simulink model "UAM_decentralized"  (R2024b)
settings: Solver=VariableStepAuto  StartTime=0.0  StopTime=20  FixedStep=Ts  RelTol=1e-3
InitFcn:
  | UAM_initialization
values from neighbouring files (symbols this model uses):
  eta_b_dot_init = [0;0;0]    [UAM_initialization.m]
  eta_b_init = [0;0;psi0]    [UAM_initialization.m]
  H_b = sym('H_b', [3 3], 'real')    [C_matrix.m]    (also in UAM_initialization.m = diag([1.24, 1.24, 2.48]))
  H_l1 = sym('H_l1', [3 3], 'real')    [C_matrix.m]    (also in C_matrix_manipulator.m; UAM_initialization.m = diag([0, 0, 0]))
  H_l2 = sym('H_l2', [3 3], 'real')    [C_matrix.m]    (also in C_matrix_manipulator.m; UAM_initialization.m = diag([0, 0, 0.0011]))
  H_l3 = sym('H_l3', [3 3], 'real')    [C_matrix.m]    (also in C_matrix_manipulator.m; UAM_initialization.m = diag([0, 0, 1.25e-4]))
  l1 = 0.15    [UAM_initialization.m]
  l2 = 0.05    [UAM_initialization.m]
  m_b = 2.0    (= 2)    [UAM_initialization.m]
  m_l1 = 0    [UAM_initialization.m]
  m_l2 = 0.049    [UAM_initialization.m]
  m_l3 = 0.05    [UAM_initialization.m]
  offset = 0.1    [UAM_initialization.m]
  p_b_dot_init = lin_vel_0'    [UAM_initialization.m]
  p_b_init = pos_0'    [UAM_initialization.m]
  q_dot_init = zeros(3,1)    [UAM_initialization.m]
  q_init = [-pi/2; 0; pi/2]    [UAM_initialization.m]
  Ts = 0.001    [UAM_initialization.m]
undefined symbols (not defined in the file or in its folder): DiscIntNeverNeededParam
libraries: cstblocks x3, simulink x2, simulink_extras x1
settings Model: Creator=giuli  LastModifiedBy=giuli

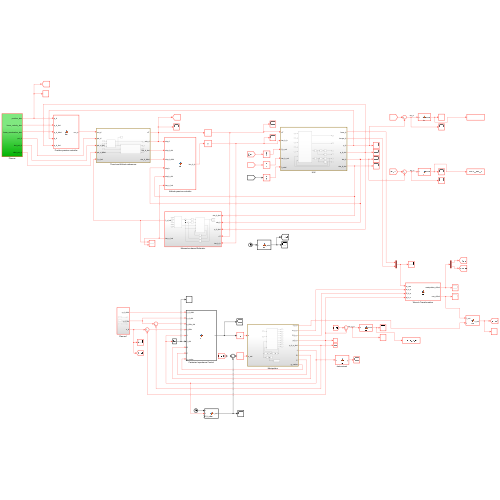
[thumbnail: Simulink's stored preview of the top-level diagram]
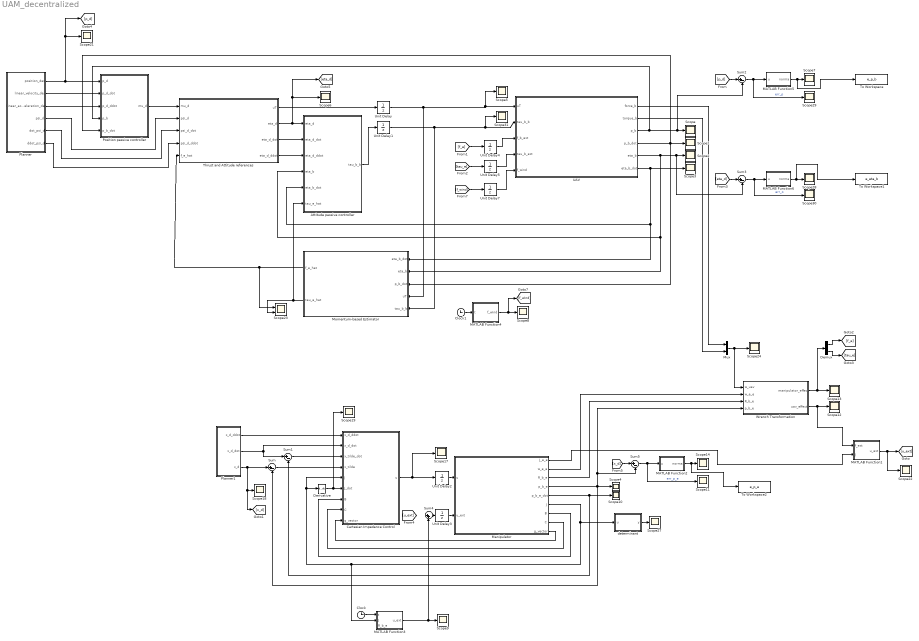
== system UAM_decentralized ==
  Attitude passive controller : MATLAB Function  TreatAsAtomicUnit=on
  Cartesian Impedance Control : MATLAB Function  TreatAsAtomicUnit=on
  Clock : Clock
      settings: Decimation=100
  Clock1 : Clock
      settings: Decimation=100
  Demux : Demux  Outputs=[3 3]
  Derivative : Derivative
  MATLAB Function1 : MATLAB Function  TreatAsAtomicUnit=on
  MATLAB Function2 : MATLAB Function  TreatAsAtomicUnit=on
  MATLAB Function3 : MATLAB Function  TreatAsAtomicUnit=on
  MATLAB Function4 : MATLAB Function  TreatAsAtomicUnit=on
  MATLAB Function5 : MATLAB Function  TreatAsAtomicUnit=on
  MATLAB Function6 : MATLAB Function  TreatAsAtomicUnit=on
  Manipulator : Subsystem
  Momentum-based Estimator : Subsystem
  Mux : Mux  Inputs=[3 3]
  Planner : Subsystem
  Planner1 : Subsystem
  Position passive controller : MATLAB Function  TreatAsAtomicUnit=on
  Scope{,1..14,17..19,21..22,24,27..31} (26 alike) : Scope
  Scope23 : Scope  NumInputPorts=2
  Sum{,1..3,5} (5 alike) : Sum  Inputs=|+-
  Sum4 : Sum  Inputs=|++
  Thrust and Attitude references : Subsystem
  To Workspace : ToWorkspace  VariableName=e_p_b  SampleTime=-1
  To Workspace1 : ToWorkspace  VariableName=e_eta_b  SampleTime=-1
  To Workspace2 : ToWorkspace  VariableName=e_p_e  SampleTime=-1
  UAV : Subsystem
  Unit Delay : UnitDelay  InitialCondition=m_b*9.81  SampleTime=Ts  HasFrameUpgradeWarning=on
  Unit Delay{1..5} (5 alike) : UnitDelay  SampleTime=Ts  HasFrameUpgradeWarning=on
  Unit Delay7 : UnitDelay  SampleTime=-1  HasFrameUpgradeWarning=on
  Wrench Transformation : MATLAB Function  TreatAsAtomicUnit=on
  determinant : MATLAB Function  TreatAsAtomicUnit=on
  wires:
  Attitude passive controller/1(tau_b_b) -> Unit Delay1/1
  [f_e] -> Unit Delay4/1
  [tau_e] -> Unit Delay5/1
  Thrust and Attitude references/4(eta_d_ddot) -> Attitude passive controller/3(eta_d_ddot)
  Thrust and Attitude references/1(uT) -> Unit Delay/1
  Thrust and Attitude references/3(eta_d_dot) -> Attitude passive controller/2(eta_d_dot)
  Thrust and Attitude references/2(eta_d) -> Attitude passive controller/1(eta_d), Scope6/1, [eta_d]
  Position passive controller/1(mu_d) -> Thrust and Attitude references/1(mu_d)
  Planner/1(position_des) -> Scope21/1, [p_d], Position passive controller/1(p_d)
  Planner/2(linear_velocity_des) -> Position passive controller/2(p_d_dot)
  Planner/3(linear_acceleration_des) -> Position passive controller/3(p_d_ddot)
  Planner/4(psi_d) -> Thrust and Attitude references/2(psi_d)
  Planner/5(dot_psi_d) -> Thrust and Attitude references/3(psi_d_dot)
  Planner/6(ddot_psi_d) -> Thrust and Attitude references/4(psi_d_ddot)
  Momentum-based Estimator/2(tau_e_hat) -> Scope23/2, Attitude passive controller/6(tau_e_hat)
  Momentum-based Estimator/1(f_e_hat) -> Thrust and Attitude references/5(f_e_hat), Scope23/1
  UAV/6(eta_b_dot) -> Attitude passive controller/5(eta_b_dot), Momentum-based Estimator/1(eta_b_dot), Scope3/1
  UAV/5(eta_b) -> Sum3/2, Scope2/1, Attitude passive controller/4(eta_b), Momentum-based Estimator/2(eta_b)
  UAV/4(p_b_dot) -> Position passive controller/5(p_b_dot), Scope1/1, Momentum-based Estimator/3(p_b_dot)
  UAV/3(p_b) -> Position passive controller/4(p_b), Scope/1, Sum2/2
  Sum/1 -> Cartesian Impedance Control/4(x_tilde)
  Manipulator/9(g_vector) -> Cartesian Impedance Control/9(g_vector)
  MATLAB Function3/1(u_ext) -> Sum4/2, Scope9/1
  Manipulator/8(C) -> Cartesian Impedance Control/8(C)
  Sum1/1 -> Cartesian Impedance Control/3(x_tilde_dot)
  Unit Delay2/1 -> Manipulator/1(u)
  Clock/1 -> MATLAB Function3/1(t)
  Manipulator/4(p_b_e) -> Wrench Transformation/4(p_b_e), Sum5/2, Scope4/1, Sum/2
  Manipulator/5(p_b_e_dot) -> Scope10/1, Sum1/2
  Manipulator/7(B) -> Cartesian Impedance Control/7(B)
  Derivative/1 -> Scope19/1, Cartesian Impedance Control/6(J_dot)
  MATLAB Function1/1(u_ext) -> [u_ext], Scope22/1
  Demux/1 -> [f_e]
  Unit Delay4/1 -> UAV/3(f_b_ext)
  UAV/1(force_b) -> Mux/1
  UAV/2(torque_b) -> Mux/2
  Manipulator/6(J) -> determinant/1(u), Derivative/1, Cartesian Impedance Control/5(J), MATLAB Function3/2(J)
  Planner1/3(x_d) -> [x_d], Scope18/1, Sum/1
  Planner1/2(x_d_dot) -> Sum1/1, Cartesian Impedance Control/2(x_d_dot)
  Planner1/1(x_d_ddot) -> Cartesian Impedance Control/1(x_d_ddot)
  Cartesian Impedance Control/1(u) -> Unit Delay2/1, Scope17/1
  determinant/1(y) -> Scope27/1
  Unit Delay/1 -> Scope5/1, UAV/1(uT), Momentum-based Estimator/4(uT)
  Unit Delay1/1 -> Scope31/1, UAV/2(tau_b_b), Momentum-based Estimator/5(tau_b_b)
  Wrench Transformation/1(manipulator_effect) -> Demux/1, Scope13/1
  Wrench Transformation/2(uav_effect) -> MATLAB Function1/1(f_ext), Scope12/1
  Demux/2 -> [tau_e]
  Unit Delay5/1 -> UAV/4(tau_b_ext)
  [p_d] -> Sum2/1
  Sum2/1 -> Scope29/1, MATLAB Function5/1(u)  "err_p"
  MATLAB Function5/1(norma) -> To Workspace/1, Scope7/1
  MATLAB Function6/1(norma) -> To Workspace1/1, Scope28/1
  Sum3/1 -> Scope30/1, MATLAB Function6/1(u)  "err_o"
  [eta_d] -> Sum3/1
  [x_d] -> Sum5/1
  Sum5/1 -> Scope11/1, MATLAB Function2/1(u)  "err_p_e"
  MATLAB Function2/1(norma) -> To Workspace2/1, Scope14/1
  Manipulator/2(w_e_e) -> Wrench Transformation/2(w_e_e)
  Manipulator/3(R_b_e) -> Wrench Transformation/3(R_b_e)
  Manipulator/1(J_e_e) -> MATLAB Function1/2(J)
  Mux/1 -> Wrench Transformation/1(w_uav), Scope24/1
  Clock1/1 -> MATLAB Function4/1(t)
  MATLAB Function4/1(f_wind) -> [f_wind], Scope8/1
  Sum4/1 -> Unit Delay3/1
  Unit Delay7/1 -> UAV/5(f_wind)
  [f_wind] -> Unit Delay7/1
  Unit Delay3/1 -> Manipulator/2(u_ext)

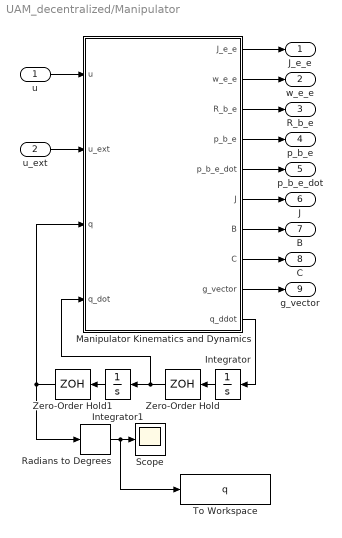
== system UAM_decentralized/Manipulator ==
  u : Inport
  u_ext : Inport  Port=2
  Integrator : Integrator  InitialCondition=q_dot_init
  Integrator1 : Integrator  InitialCondition=q_init
  Manipulator Kinematics and Dynamics : MATLAB Function  TreatAsAtomicUnit=on
  Radians to Degrees : simulink_extras/Transformations/Radians to Degrees
  Scope : Scope
  To Workspace : ToWorkspace  VariableName=q  SampleTime=-1
  Zero-Order Hold : ZeroOrderHold  SampleTime=Ts
  Zero-Order Hold1 : ZeroOrderHold  SampleTime=Ts
  J_e_e : Outport
  w_e_e : Outport  Port=2
  R_b_e : Outport  Port=3
  p_b_e : Outport  Port=4
  p_b_e_dot : Outport  Port=5
  J : Outport  Port=6
  B : Outport  Port=7
  C : Outport  Port=8
  g_vector : Outport  Port=9
  wires:
  u_ext/1 -> Manipulator Kinematics and Dynamics/2(u_ext)
  Manipulator Kinematics and Dynamics/9(g_vector) -> g_vector/1
  u/1 -> Manipulator Kinematics and Dynamics/1(u)
  Manipulator Kinematics and Dynamics/6(J) -> J/1
  Manipulator Kinematics and Dynamics/7(B) -> B/1
  Manipulator Kinematics and Dynamics/8(C) -> C/1
  Manipulator Kinematics and Dynamics/3(R_b_e) -> R_b_e/1
  Manipulator Kinematics and Dynamics/4(p_b_e) -> p_b_e/1
  Manipulator Kinematics and Dynamics/5(p_b_e_dot) -> p_b_e_dot/1
  Integrator/1 -> Zero-Order Hold/1
  Manipulator Kinematics and Dynamics/10(q_ddot) -> Integrator/1
  Integrator1/1 -> Zero-Order Hold1/1
  Radians to Degrees/1 -> To Workspace/1, Scope/1
  Zero-Order Hold1/1 -> Manipulator Kinematics and Dynamics/3(q), Radians to Degrees/1
  Zero-Order Hold/1 -> Integrator1/1, Manipulator Kinematics and Dynamics/4(q_dot)
  Manipulator Kinematics and Dynamics/2(w_e_e) -> w_e_e/1
  Manipulator Kinematics and Dynamics/1(J_e_e) -> J_e_e/1

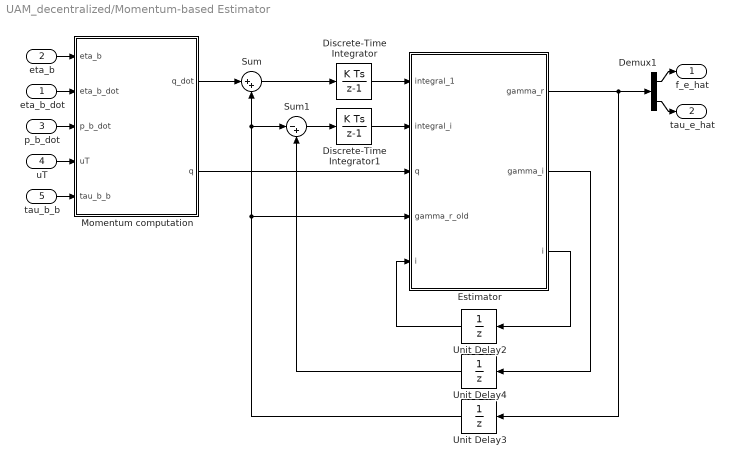
== system UAM_decentralized/Momentum-based Estimator ==
  eta_b_dot : Inport
  eta_b : Inport  Port=2
  p_b_dot : Inport  Port=3
  uT : Inport  Port=4
  tau_b_b : Inport  Port=5
  Demux1 : Demux  Outputs=[3 3]
  Discrete-Time Integrator : DiscreteIntegrator  SampleTime=Ts  ICPrevOutput=DiscIntNeverNeededParam  ICPrevScaledInput=DiscIntNeverNeededParam
  Discrete-Time Integrator1 : DiscreteIntegrator  SampleTime=Ts  ICPrevOutput=DiscIntNeverNeededParam  ICPrevScaledInput=DiscIntNeverNeededParam
  Estimator : MATLAB Function  TreatAsAtomicUnit=on
  Momentum computation : MATLAB Function  TreatAsAtomicUnit=on
  Sum : Sum  Inputs=|++
  Sum1 : Sum  Inputs=|-+
  Unit Delay2 : UnitDelay  SampleTime=-1  HasFrameUpgradeWarning=on
  Unit Delay3 : UnitDelay  SampleTime=-1  HasFrameUpgradeWarning=on
  Unit Delay4 : UnitDelay  SampleTime=-1  HasFrameUpgradeWarning=on
  f_e_hat : Outport
  tau_e_hat : Outport  Port=2
  wires:
  Discrete-Time Integrator/1 -> Estimator/1(integral_1)
  Unit Delay2/1 -> Estimator/5("i ")
  Discrete-Time Integrator1/1 -> Estimator/2(integral_i)
  Unit Delay4/1 -> Sum1/2
  eta_b/1 -> Momentum computation/1(eta_b)
  Demux1/1 -> f_e_hat/1
  Estimator/1(gamma_r) -> Demux1/1, Unit Delay3/1
  Estimator/3(i) -> Unit Delay2/1
  Unit Delay3/1 -> Estimator/4(gamma_r_old), Sum/2, Sum1/1
  Estimator/2(gamma_i) -> Unit Delay4/1
  Sum1/1 -> Discrete-Time Integrator1/1
  Sum/1 -> Discrete-Time Integrator/1
  Momentum computation/1(q_dot) -> Sum/1
  eta_b_dot/1 -> Momentum computation/2(eta_b_dot)
  p_b_dot/1 -> Momentum computation/3(p_b_dot)
  uT/1 -> Momentum computation/4(uT)
  tau_b_b/1 -> Momentum computation/5(tau_b_b)
  Demux1/2 -> tau_e_hat/1
  Momentum computation/2(q) -> Estimator/3(q)

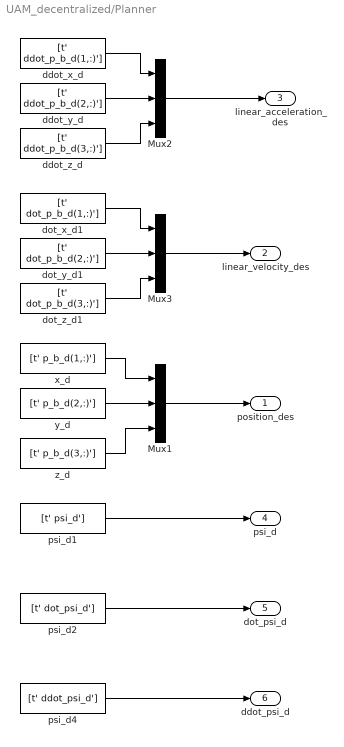
== system UAM_decentralized/Planner ==
  Mux1 : Mux  Inputs=3
  Mux2 : Mux  Inputs=3
  Mux3 : Mux  Inputs=3
  ddot_x_d : FromWorkspace  VariableName=[t' ddot_p_b_d(1,:)']  SampleTime=Ts
  ddot_y_d : FromWorkspace  VariableName=[t' ddot_p_b_d(2,:)']  SampleTime=Ts
  ddot_z_d : FromWorkspace  VariableName=[t' ddot_p_b_d(3,:)']  SampleTime=Ts
  dot_x_d1 : FromWorkspace  VariableName=[t' dot_p_b_d(1,:)']  SampleTime=Ts
  dot_y_d1 : FromWorkspace  VariableName=[t' dot_p_b_d(2,:)']  SampleTime=Ts
  dot_z_d1 : FromWorkspace  VariableName=[t' dot_p_b_d(3,:)']  SampleTime=Ts
  psi_d1 : FromWorkspace  VariableName=[t' psi_d']  SampleTime=Ts
  psi_d2 : FromWorkspace  VariableName=[t' dot_psi_d']  SampleTime=Ts
  psi_d4 : FromWorkspace  VariableName=[t' ddot_psi_d']  SampleTime=Ts
  x_d : FromWorkspace  VariableName=[t' p_b_d(1,:)']  SampleTime=Ts
  y_d : FromWorkspace  VariableName=[t' p_b_d(2,:)']  SampleTime=Ts
  z_d : FromWorkspace  VariableName=[t' p_b_d(3,:)']  SampleTime=Ts
  position_des : Outport
  linear_velocity_des : Outport  Port=2
  linear_acceleration_des : Outport  Port=3
  psi_d : Outport  Port=4
  dot_psi_d : Outport  Port=5
  ddot_psi_d : Outport  Port=6
  wires:
  y_d/1 -> Mux1/2
  z_d/1 -> Mux1/3
  x_d/1 -> Mux1/1
  ddot_y_d/1 -> Mux2/2
  ddot_z_d/1 -> Mux2/3
  ddot_x_d/1 -> Mux2/1
  Mux2/1 -> linear_acceleration_des/1
  Mux1/1 -> position_des/1
  dot_y_d1/1 -> Mux3/2
  dot_z_d1/1 -> Mux3/3
  dot_x_d1/1 -> Mux3/1
  Mux3/1 -> linear_velocity_des/1
  psi_d1/1 -> psi_d/1
  psi_d2/1 -> dot_psi_d/1
  psi_d4/1 -> ddot_psi_d/1

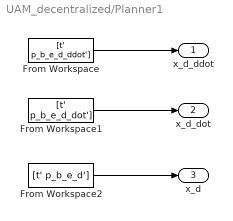
== system UAM_decentralized/Planner1 ==
  From Workspace : FromWorkspace  VariableName=[t' p_b_e_d_ddot']  SampleTime=Ts
  From Workspace1 : FromWorkspace  VariableName=[t' p_b_e_d_dot']  SampleTime=Ts
  From Workspace2 : FromWorkspace  VariableName=[t' p_b_e_d']  SampleTime=Ts
  x_d_ddot : Outport
  x_d_dot : Outport  Port=2
  x_d : Outport  Port=3
  wires:
  From Workspace/1 -> x_d_ddot/1
  From Workspace2/1 -> x_d/1
  From Workspace1/1 -> x_d_dot/1

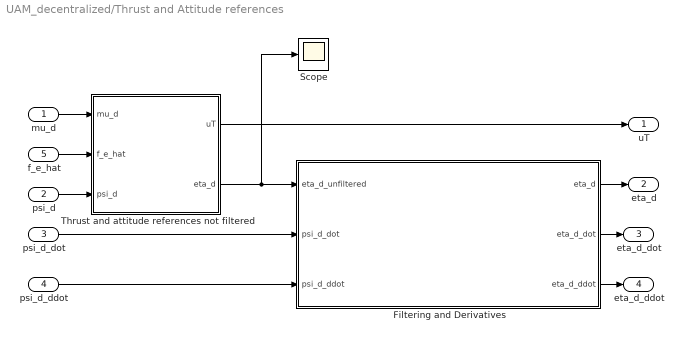
== system UAM_decentralized/Thrust and Attitude references ==
  mu_d : Inport
  psi_d : Inport  Port=2
  psi_d_dot : Inport  Port=3
  psi_d_ddot : Inport  Port=4
  f_e_hat : Inport  Port=5
  Filtering and Derivatives : Subsystem
  Scope : Scope
  Thrust and attitude references not filtered : MATLAB Function  TreatAsAtomicUnit=on
  uT : Outport
  eta_d : Outport  Port=2
  eta_d_dot : Outport  Port=3
  eta_d_ddot : Outport  Port=4
  wires:
  Thrust and attitude references not filtered/2(eta_d) -> Scope/1, Filtering and Derivatives/1(eta_d_unfiltered)
  psi_d_dot/1 -> Filtering and Derivatives/2(psi_d_dot)
  Filtering and Derivatives/3(eta_d_ddot) -> eta_d_ddot/1
  mu_d/1 -> Thrust and attitude references not filtered/1(mu_d)
  Filtering and Derivatives/1(eta_d) -> eta_d/1
  psi_d_ddot/1 -> Filtering and Derivatives/3(psi_d_ddot)
  Filtering and Derivatives/2(eta_d_dot) -> eta_d_dot/1
  f_e_hat/1 -> Thrust and attitude references not filtered/2(f_e_hat)
  psi_d/1 -> Thrust and attitude references not filtered/3(psi_d)
  Thrust and attitude references not filtered/1(uT) -> uT/1

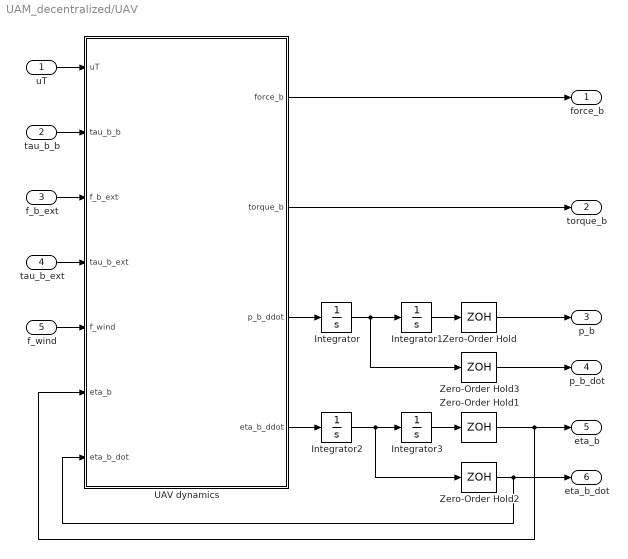
== system UAM_decentralized/UAV ==
  uT : Inport
  tau_b_b : Inport  Port=2
  f_b_ext : Inport  Port=3
  tau_b_ext : Inport  Port=4
  f_wind : Inport  Port=5
  Integrator : Integrator  InitialCondition=p_b_dot_init
  Integrator1 : Integrator  InitialCondition=p_b_init
  Integrator2 : Integrator  InitialCondition=eta_b_dot_init
  Integrator3 : Integrator  InitialCondition=eta_b_init
  UAV dynamics : MATLAB Function  TreatAsAtomicUnit=on
  Zero-Order Hold{,1..3} (4 alike) : ZeroOrderHold  SampleTime=Ts
  force_b : Outport
  torque_b : Outport  Port=2
  p_b : Outport  Port=3
  p_b_dot : Outport  Port=4
  eta_b : Outport  Port=5
  eta_b_dot : Outport  Port=6
  wires:
  Integrator2/1 -> Integrator3/1, Zero-Order Hold2/1
  Zero-Order Hold2/1 -> eta_b_dot/1, UAV dynamics/7(eta_b_dot)
  Integrator3/1 -> Zero-Order Hold1/1
  tau_b_ext/1 -> UAV dynamics/4(tau_b_ext)
  Zero-Order Hold3/1 -> p_b_dot/1
  Integrator/1 -> Integrator1/1, Zero-Order Hold3/1
  UAV dynamics/3(p_b_ddot) -> Integrator/1
  uT/1 -> UAV dynamics/1(uT)
  UAV dynamics/4(eta_b_ddot) -> Integrator2/1
  Integrator1/1 -> Zero-Order Hold/1
  Zero-Order Hold1/1 -> eta_b/1, UAV dynamics/6(eta_b)
  Zero-Order Hold/1 -> p_b/1
  tau_b_b/1 -> UAV dynamics/2(tau_b_b)
  f_b_ext/1 -> UAV dynamics/3(f_b_ext)
  UAV dynamics/1(force_b) -> force_b/1
  UAV dynamics/2(torque_b) -> torque_b/1
  f_wind/1 -> UAV dynamics/5(f_wind)

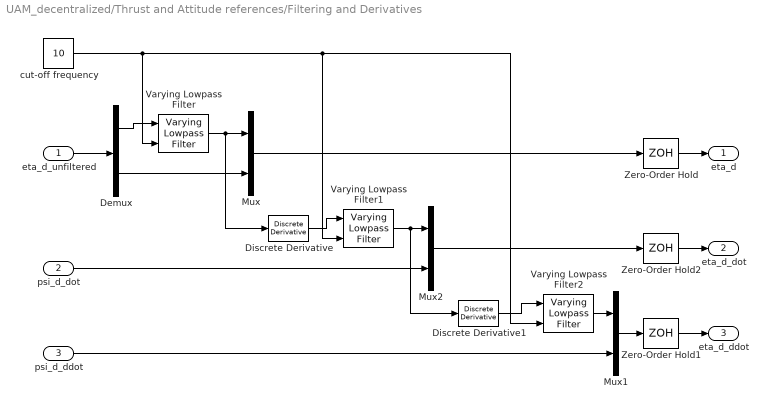
== system UAM_decentralized/Thrust and Attitude references/Filtering and Derivatives ==
  eta_d_unfiltered : Inport
  psi_d_dot : Inport  Port=2
  psi_d_ddot : Inport  Port=3
  Demux : Demux  Outputs=[2 1]
  Discrete Derivative : simulink/Discrete/Discrete Derivative  gainval=1.0  ICPrevScaledInput=0.0  OutMin=[]  OutMax=[]  OutDataType=fixdt(1, 16)  OutScaling=2^-10  DoSatur=off
  Discrete Derivative1 : simulink/Discrete/Discrete Derivative  gainval=1.0  ICPrevScaledInput=0.0  OutMin=[]  OutMax=[]  OutDataType=fixdt(1, 16)  OutScaling=2^-10  DoSatur=off
  Mux : Mux  Inputs=[2 1]
  Mux1 : Mux  Inputs=[2 1]
  Mux2 : Mux  Inputs=[2 1]
  Varying Lowpass Filter : cstblocks/Linear Parameter Varying/Varying Lowpass Filter  N=1
  Varying Lowpass Filter1 : cstblocks/Linear Parameter Varying/Varying Lowpass Filter  N=1
  Varying Lowpass Filter2 : cstblocks/Linear Parameter Varying/Varying Lowpass Filter  N=1
  Zero-Order Hold : ZeroOrderHold  SampleTime=Ts
  Zero-Order Hold1 : ZeroOrderHold  SampleTime=Ts
  Zero-Order Hold2 : ZeroOrderHold  SampleTime=Ts
  cut-off frequency : Constant  Value=10
  eta_d : Outport
  eta_d_dot : Outport  Port=2
  eta_d_ddot : Outport  Port=3
  wires:
  Mux/1 -> Zero-Order Hold/1
  Mux1/1 -> Zero-Order Hold1/1
  Mux2/1 -> Zero-Order Hold2/1
  eta_d_unfiltered/1 -> Demux/1
  psi_d_ddot/1 -> Mux1/2
  Varying Lowpass Filter1/1 -> Discrete Derivative1/1, Mux2/1
  Demux/2 -> Mux/2
  Demux/1 -> Varying Lowpass Filter/1
  Varying Lowpass Filter/1 -> Discrete Derivative/1, Mux/1
  cut-off frequency/1 -> Varying Lowpass Filter/2, Varying Lowpass Filter2/2, Varying Lowpass Filter1/2
  psi_d_dot/1 -> Mux2/2
  Discrete Derivative/1 -> Varying Lowpass Filter1/1
  Discrete Derivative1/1 -> Varying Lowpass Filter2/1
  Varying Lowpass Filter2/1 -> Mux1/1
  Zero-Order Hold/1 -> eta_d/1
  Zero-Order Hold1/1 -> eta_d_ddot/1
  Zero-Order Hold2/1 -> eta_d_dot/1

== matlab function UAM_decentralized/Momentum-based Estimator/Momentum computation ==
  data: q_dot output; eta_b input; q output; eta_b_dot input; p_b_dot input; uT input; tau_b_b input; m_b parameter; H_b parameter
function [q_dot,q] = fcn(eta_b, eta_b_dot, p_b_dot, uT, tau_b_b,  m_b, H_b)

% parameters
g = 9.81;
e3 = [0;0;1];

%% Extracting variables
% Euler angles
phi = eta_b(1);    % Roll angle
theta = eta_b(2);  % Pitch angle
psi = eta_b(3);    % Yaw angle

phi_dot = eta_b_dot(1);   
theta_dot = eta_b_dot(2);  
%psi_dot = eta_b_dot(3);    

%% Rotation Matrices and Angular Velocity Mapping
% Individual Rotation Matrices
% Rotation about X-axis (Roll)
Rx = [1,           0,          0;
      0, cos(phi), -sin(phi);
      0, sin(phi),  cos(phi)];

% Rotation about Y-axis (Pitch)
Ry = [cos(theta),  0, sin(theta);
      0,           1,          0;
     -sin(theta),  0, cos(theta)];

% Rotation about Z-axis (Yaw)
Rz = [cos(psi), -sin(psi), 0;
      sin(psi),  cos(psi), 0;
      0,         0,         1];

% Combined Rotation Matrix R_b (from UAV body frame to Inertial frame)
% Using Z-Y-X Euler angle convention (Yaw-Pitch-Roll)
R_b = Rz * Ry * Rx;

% mapping between time derivative of eta_b into UAV angular velocity omega_b_b expressed wrt Sigma_b
Q = [   1     0           -sin(theta);
        0     cos(phi)    cos(theta)*sin(phi);
        0     -sin(phi)   cos(theta)*cos(phi)];

Q_dot = [ 0,     0,                     -cos(theta)*theta_dot;
          0,    -sin(phi)*phi_dot,     -sin(theta)*sin(phi)*theta_dot + cos(theta)*cos(phi)*phi_dot;
          0,    -cos(phi)*phi_dot,     -sin(theta)*cos(phi)*theta_dot - cos(theta)*sin(phi)*phi_dot ];

%% Dynamic Matrices
M = Q' * H_b * Q;    % inertia matrix
C = Q' * skew(Q * eta_b_dot) * H_b * Q + Q' * H_b * Q_dot;    % Coriolis matrix

%% Generalized momentum q
q = [m_b * p_b_dot;
    M * eta_b_dot];

q_dot = [m_b*g*e3 - uT*R_b*e3;
        C'*eta_b_dot + Q'*tau_b_b];

end

function S = skew(v)
if(numel(v)~= 1)
S= [0 -v(3) v(2); 
    v(3) 0 -v(1);
    -v(2) v(1) 0];
else
S= zeros(3);
end
end

== matlab function UAM_decentralized/Momentum-based Estimator/Estimator ==
  data: gamma_r output; integral_1 input; gamma_i output; integral_i input; q input; gamma_r_old input; i output; i input; K parameter
function [gamma_r, gamma_i, i] = fcn(integral_1, integral_i, q, gamma_r_old,i,  K)

r = 2;

gamma_i = zeros(6,1);
gamma_r = gamma_r_old;

if i == 0   % first step
    i = i+1;
    gamma_i = K(1) * (q - integral_1);
else 
    i = i+1;
    gamma_i = K(i) * integral_i;
    if i == r
        gamma_r = gamma_i;  % final step
        i = 0;  % to reset
    end
end

== matlab function UAM_decentralized/MATLAB Function3 ==
  data: t input; J input; u_ext output; R_b_e input
function u_ext = fcn(t,J,R_b_e)
% A = 1;
% omega = pi/2;
% 
% if t <= 10
%     wind = A*sin(omega*t);
% 
%     if wind >= 0
%         f_ext = [wind; zeros(2,1)];
%     else
%         f_ext = zeros(3,1);
%     end
% else
%     f_ext = zeros(3,1);
% end
% 
% f_ext = R_b_e * [0; 0; 1];

f_wall = [-0.5;0;0];
u_ext = J' * f_wall;

== matlab function UAM_decentralized/MATLAB Function4 ==
  data: t input; f_wind output
function f_wind = fcn(t)
A = 1;
omega = pi/2;

if t <= 10
    wind = A*sin(omega*t);

    if wind >= 0
        f_ext = [wind; zeros(2,1)];
    else
        f_ext = zeros(3,1);
    end
else
    f_ext = zeros(3,1);
end

f_wind = [f_ext(1:3)]; 


% % u_ext = J' * f_ext;

== matlab function UAM_decentralized/Manipulator/Manipulator Kinematics and Dynamics ==
  data: J_e_e output; w_e_e output; R_b_e output; p_b_e output; p_b_e_dot output; J output; B output; C output; g_vector output; u input; u_ext input; q input; q_ddot output; q_dot input; m_l1 parameter; m_l2 parameter; m_l3 parameter; l1 parameter; l2 parameter; H_l1 parameter; H_l2 parameter; H_l3 parameter; offset parameter
function [J_e_e,w_e_e,R_b_e, p_b_e,p_b_e_dot,  J,B,C,g_vector,  q_ddot] = fcn(u, u_ext, q,q_dot, m_l1, m_l2, m_l3, l1, l2, H_l1, H_l2, H_l3, offset) % m_b, H_b

% Parameters
g = 9.81;       % gravity acceleration value
e3 = [0;0;1];   % selecting vector

%% State Variables from Generalized Joints Vector (csi)
% % Extracting components of the generalized state vector 'csi'
% p_b = csi(1:3);    % Position of UAV body frame origin in inertial frame
% eta_b = csi(4:6);  % Euler angles (Yaw, Pitch, Roll) of UAV body frame
% q = csi(7:9);      % Manipulator joint angles
% 
% % Euler angles
% phi = eta_b(1);    % Roll angle
% theta = eta_b(2);  % Pitch angle
% psi = eta_b(3);    % Yaw angle

%% UAV Kinematics: Rotation Matrices and Angular Velocity Mapping
% % Individual Rotation Matrices
% % Rotation about X-axis (Roll)
% Rx = [1,           0,          0;
%       0, cos(phi), -sin(phi);
%       0, sin(phi),  cos(phi)];
% 
% % Rotation about Y-axis (Pitch)
% Ry = [cos(theta),  0, sin(theta);
%       0,           1,          0;
%      -sin(theta),  0, cos(theta)];
% 
% % Rotation about Z-axis (Yaw)
% Rz = [cos(psi), -sin(psi), 0;
%       sin(psi),  cos(psi), 0;
%       0,         0,         1];
% 
% % Combined Rotation Matrix R_b (from UAV body frame to Inertial frame)
% % Using Z-Y-X Euler angle convention (Yaw-Pitch-Roll)
% R_b = Rz * Ry * Rx;
% 
% % mapping between time derivative of eta_b into UAV angular velocity omega_b_b expressed wrt Sigma_b
% Q = [   1     0           -sin(theta);
%         0     cos(phi)    cos(theta)*sin(phi);
%         0     -sin(phi)   cos(theta)*cos(phi)];    % It's easier to compute first Q
% 
% % T_b matrix: Maps Euler angle rates (phi_dot) to body angular velocity (omega_b)
% % omega_b = T_b * phi_dot
% T_b = R_b * Q;        % it's easier this way
% 
% % Q = R_b' * T_b;     
% 
% % Ab: Homogeneous transformation matrix from Inertial frame to UAV Body frame
% A_b = [R_b,   p_b;
%       0 0 0, 1];


%% Manipulator Direct Kinematics (Relative to UAV Body Frame)
% Static Transformation to take into account the offset between UAV and Manipulator

R_b_0 = [1,           0,          0;
        0, cos(pi/2), -sin(pi/2);
        0, sin(pi/2),  cos(pi/2)];  % rotation of pi/2 about x-axis


T_b_0 = [   R_b_0, [0;0;-offset];      % translation along zb
            0,   0,   0,   1];

% D-H parameters for the manipulator
a = [0, l1, l2];
d = [0, 0, 0];
alpha = [pi/2, -pi/2, 0];

% Standard DH transformation matrix A(alpha, a, d, theta) - here theta is q_i
DH_matrix = @(alpha_i, a_i, d_i, q_i) ...
    [cos(q_i), -sin(q_i)*cos(alpha_i),  sin(q_i)*sin(alpha_i),  a_i*cos(q_i);
     sin(q_i),  cos(q_i)*cos(alpha_i), -cos(q_i)*sin(alpha_i),  a_i*sin(q_i);
     0,         sin(alpha_i),          cos(alpha_i),           d_i;
     0,         0,                     0,                      1];

A_0_1 = DH_matrix(alpha(1), a(1), d(1), q(1));
A_1_2 = DH_matrix(alpha(2), a(2), d(2), q(2));
A_2_3 = DH_matrix(alpha(3), a(3), d(3), q(3));

% Transformations from manipulator base frame (Frame 0) to each link frame
T_0_0 = eye(4); % Transformation from Frame 0 to Frame 0
T_0_1 = A_0_1;  % Transformation from Frame 0 to Frame 1
T_0_2 = A_0_1 * A_1_2; % Transformation from Frame 0 to Frame 2
T_0_3 = A_0_1 * A_1_2 * A_2_3; % Transformation from Frame 0 to Frame 3

R_0_0 = T_0_0(1:3, 1:3); p_0_0 = T_0_0(1:3, 4);
R_0_1 = T_0_1(1:3, 1:3); p_0_1 = T_0_1(1:3, 4);
R_0_2 = T_0_2(1:3, 1:3); p_0_2 = T_0_2(1:3, 4);

% Rotation about the y-axis
R_3_e = [cos(pi/2),  0, sin(pi/2);
        0,           1,          0;
        -sin(pi/2),  0, cos(pi/2)];
% To align the z-axis to the approach axis
T_3_e = [R_3_e,         zeros(3,1);
         zeros(1,3),    1];

T_0_e = T_0_3 * T_3_e;

p_0_e = T_0_e(1:3, 4);
R_0_e = T_0_e(1:3, 1:3);

% Direct kinematic of the Manipulator from UAV body frame to end-effector frame
A_b_e = T_b_0 * T_0_3 * T_3_e;

% Extract position of end-effector frame origin in UAV body frame (p_b_e)
% p_e^b is position vector of the origin of end-effector frame wrt Sigma_b 
p_b_e = A_b_e(1:3, 4);

R_b_e = A_b_e(1:3, 1:3);

%% Absolute Pose of the End-Effector
% % A_e: Absolute homogeneous transformation matrix of the end-effector (in Inertial frame)
% A_e = A_b * A_b_e;
% 
% R_e = A_e(1:3, 1:3);
% 
% % Extract p_e (position of end-effector in inertial frame)
% p_e = A_e(1:3, 4); % This is p_e from x = [p_b^T, eta_b^T, p_e^T]^T 
% 
% x = [p_b; eta_b; p_e];

%% Manipulator Jacobian (in manipulator 0 frame)
% For revolute joints
% JPi = z_{i-1} X (p_e - p_{i-1})
% JOi = z_{i-1}

% z_{i-1} is the third column of the rotation matrix R_0_{i-1}
z_0 = R_0_0(:, 3);
z_1 = R_0_1(:, 3);
z_2 = R_0_2(:, 3);

% Manipulator Translational Jacobian (J_P_0_e) for End-Effector in Frame 0
J_P_0_e = zeros(3,3);
J_P_0_e(:,1) = skew(z_0) * (p_0_e - p_0_0);
J_P_0_e(:,2) = skew(z_1) * (p_0_e - p_0_1);
J_P_0_e(:,3) = skew(z_2) * (p_0_e - p_0_2);

% Manipulator Rotational Jacobian (J_O_0_e) for End-Effector in Frame 0
J_O_0_e = zeros(3,3);
J_O_0_e(:,1) = z_0;
J_O_0_e(:,2) = z_1;
J_O_0_e(:,3) = z_2;

%% General System Jacobian (J, 9x9 matrix mapping csi_dot to x_dot)
% csi_dot = [p_b_dot; eta_b_dot; q_dot]
% x_dot = [p_b_dot; eta_b_dot; p_e_dot]
% J = zeros(9,9);

% % --- Row Block 1 (for p_b_dot = p_b_dot) ---
% J(1:3, 1:3) = eye(3);
% J(1:3, 4:6) = zeros(3); % No dependence on eta_b_dot
% J(1:3, 7:9) = zeros(3); % No dependence on q_dot
% 
% % --- Row Block 2 (for eta_b_dot = eta_b_dot) ---
% J(4:6, 1:3) = zeros(3); % No dependence on p_b_dot
% J(4:6, 4:6) = eye(3);
% J(4:6, 7:9) = zeros(3); % No dependence on q_dot

% % --- Row Block 3 (for p_e_dot) ---
% % p_e = p_b + R_b * p_b_e
% % p_e_dot = p_b_dot + R_b_dot * p_b_e + R_b * p_b_e_dot
% 
% % R_b_dot = skew(omega_b) * R_b
% % skew(omega_b) * R_b * p_b_e = -skew(R_b * p_b_e) * omega_b     Anti-commutative property
% % Using omega_b = T_b * eta_b_dot:
% % p_e_dot = p_b_dot - skew(R_b * p_b_e) * T_b * eta_b_dot + R_b * R_b_0 * J_P_0_e * q_dot
% J(7:9, 1:3) = eye(3);                        % Coefficient of pb_dot
% J(7:9, 4:6) = -skew(R_b * p_b_e) * T_b;      % Coefficient of eta_b_dot
% J(7:9, 7:9) = R_b * R_b_0 * J_P_0_e;         % Coefficient of q_dot

% csi_dot = [q_dot]
% x_dot = [p_b_e_dot]
J = R_b_0 * J_P_0_e;

J_e_e = [R_0_e' * J_P_0_e;
         R_0_e' * J_O_0_e];
J_P_e_e = R_0_e' * J_P_0_e;

% x_dot = J * csi_dot;
p_b_e_dot = J * q_dot;

%% Link CoM Transformations and Rotations
% Computation of "p_b_li" which is the position of the center of mass of the link i with respect to UAV body frame (Sigma_b)
% Define Center of Mass (CoM) Positions in the DH's Own Frame
% Remember that the first two joints are in the same point before Link 1
% So let's call the actual Link 1 with "Link 2"
p_0_l1 = [0; 0; 0];
p_1_l2 = [l1/2; 0; 0];
p_2_l3 = [l2/2; 0; 0];

% For Link 1    (It doesn't actually exist)
p_b_0 = T_b_0(1:3, 4);
p_b_l1 = p_b_0 + R_b_0 * p_0_l1;     % Position of the CoM of Link 1 wrt Sigma_b
R_b_l1 = R_b_0;                      % Rotation matrix between the frame associated to the center of mass of the i-th link and Σb

% For Link 2
T_b_1 = T_b_0 * T_0_1;
R_b_1 = T_b_1(1:3, 1:3);
p_b_1 = T_b_1(1:3, 4);
p_b_l2 = p_b_1 + R_b_1 * p_1_l2;     % Position of the CoM of Link 2 wrt Sigma_b
R_b_l2 = R_b_1;

% For Link 2
T_b_2 = T_b_0 * T_0_2;
R_b_2 = T_b_2(1:3, 1:3);
p_b_2 = T_b_2(1:3, 4);
p_b_l3 = p_b_2 + R_b_2 * p_2_l3;     % Position of the CoM of Link 3 wrt Sigma_b
R_b_l3 = R_b_2;

%% Jacobians for Each Link's CoM (wrt Sigma_b)
% For revolute joints
% J_Pj_li = z_{j-1} X (p_com_i - p_{j-1})   % Jacobian for contribution of the first j joints to the linear motion of CoM of Link i
% J_Oj_li = z_{j-1}                         % Jacobian for contribution of the first j joints to the angular motion of CoM of Link i


% z_{j-1} is the third column of the rotation matrix R_b_{j-1}
z_0 = R_b_0(:, 3);
z_1 = R_b_1(:, 3);
z_2 = R_b_2(:, 3);

% Link 1
J_P_l1 = zeros(3,3);
J_P_l1(:,1) = skew(z_0) * (p_b_l1 - p_b_0);

J_O_l1 = zeros(3,3);
J_O_l1(:,1) = z_0;

% Link 2
J_P_l2 = zeros(3,3);
J_P_l2(:,1) = skew(z_0) * (p_b_l2 - p_b_0);
J_P_l2(:,2) = skew(z_1) * (p_b_l2 - p_b_1);

J_O_l2 = zeros(3,3);
J_O_l2(:,1) = z_0;
J_O_l2(:,2) = z_1;

% Link 3
J_P_l3 = zeros(3,3);
J_P_l3(:,1) = skew(z_0) * (p_b_l3 - p_b_0);
J_P_l3(:,2) = skew(z_1) * (p_b_l3 - p_b_1);
J_P_l3(:,3) = skew(z_2) * (p_b_l3 - p_b_2);

J_O_l3 = zeros(3,3);
J_O_l3(:,1) = z_0;
J_O_l3(:,2) = z_1;
J_O_l3(:,3) = z_2;

%% Inertia Matrix B
% % B11
% B11 = (m_b + m_l1 + m_l2 + m_l3) * eye(3);
% 
% % B22
% B22_sum_term = m_l1 * T_b' * skew(R_b * p_b_l1)' * skew(R_b * p_b_l1) * T_b + ...
%                m_l2 * T_b' * skew(R_b * p_b_l2)' * skew(R_b * p_b_l2) * T_b + ...
%                m_l3 * T_b' * skew(R_b * p_b_l3)' * skew(R_b * p_b_l3) * T_b + ...
%                Q' * R_b_l1 * H_l1 * R_b_l1' * Q + ... 
%                Q' * R_b_l2 * H_l2 * R_b_l2' * Q + ...
%                Q' * R_b_l3 * H_l3 * R_b_l3' * Q;
% B22 = Q' * H_b * Q + B22_sum_term;

% B33
B33 = (m_l1 * (J_P_l1)' * J_P_l1 + J_O_l1' * R_b_l1 * H_l1 * R_b_l1' * J_O_l1) + ...
      (m_l2 * (J_P_l2)' * J_P_l2 + J_O_l2' * R_b_l2 * H_l2 * R_b_l2' * J_O_l2) + ...
      (m_l3 * (J_P_l3)' * J_P_l3 + J_O_l3' * R_b_l3 * H_l3 * R_b_l3' * J_O_l3);

% % B12
% B12 = - (m_l1 * skew(R_b * p_b_l1) * T_b + ...
%          m_l2 * skew(R_b * p_b_l2) * T_b + ...
%          m_l3 * skew(R_b * p_b_l3) * T_b);
% B21 = B12';
% 
% % B13
% B13 = (m_l1 * R_b * J_P_l1) + (m_l2 * R_b * J_P_l2) + (m_l3 * R_b * J_P_l3);
% B31 = B13';
% 
% % B23
% B23_sum1 = Q' * R_b_l1 * H_l1 * R_b_l1' * J_O_l1 + ...
%            Q' * R_b_l2 * H_l2 * R_b_l2' * J_O_l2 + ...
%            Q' * R_b_l3 * H_l3 * R_b_l3' * J_O_l3;
% B23_sum2 = - (m_l1 * T_b' * skew(R_b * p_b_l1)' * R_b * J_P_l1 + ...
%               m_l2 * T_b' * skew(R_b * p_b_l2)' * R_b * J_P_l2 + ...
%               m_l3 * T_b' * skew(R_b * p_b_l3)' * R_b * J_P_l3);
% B23 = B23_sum1 + B23_sum2;
% B32 = B23';

% Full B
% B = [B11, B12, B13;
%      B21, B22, B23;
%      B31, B32, B33];

B = B33;

%% Gravity vector contribution g(csi)
% Partial derivative of potential energy U wrt csi
% U = m_b * g * e3' * p_b + sum(m_li * g * e3' * (p_b + R_b * p_b_li))

% % Derivative of U wrt p_b
% g_pb = ((m_b + m_l1 + m_l2 + m_l3) * g * e3')'; 
% 
% % Derivative of U wrt eta_b     (computed using symbolic toolbox)
% g_phib = zeros(3,1);
% g_phib(1) = g*cos(phi)*cos(theta)*(m_l3*(l1 + l2/2)*(sin(q(2)) - cos(pi/2)^2*sin(q(2)) + cos(pi/2)*cos(q(2))*sin(q(1)) + cos(pi/2)^2*cos(q(1))*sin(q(2))) + (l1*m_l2*cos(pi/2)*sin(q(1)))/2) - g*cos(theta)*sin(phi)*(m_l1*offset + m_l2*offset + m_l3*offset - (l1*m_l2*sin(pi/2)*sin(q(1)))/2 - l1*m_l3*sin(pi/2)*cos(q(2))*sin(q(1)) - (l2*m_l3*sin(pi/2)*cos(q(2))*sin(q(1)))/2 + l1*m_l3*cos(pi/2)*sin(pi/2)*sin(q(2)) + (l2*m_l3*cos(pi/2)*sin(pi/2)*sin(q(2)))/2 - l1*m_l3*cos(pi/2)*sin(pi/2)*cos(q(1))*sin(q(2)) - (l2*m_l3*cos(pi/2)*sin(pi/2)*cos(q(1))*sin(q(2)))/2);
% g_phib(2) = - g*cos(theta)*((l1*m_l2*cos(q(1)))/2 + l1*m_l3*cos(q(1))*cos(q(2)) + (l2*m_l3*cos(q(1))*cos(q(2)))/2 - l1*m_l3*cos(pi/2)*sin(q(1))*sin(q(2)) - (l2*m_l3*cos(pi/2)*sin(q(1))*sin(q(2)))/2) - g*cos(phi)*sin(theta)*(m_l1*offset + m_l2*offset + m_l3*offset - (l1*m_l2*sin(pi/2)*sin(q(1)))/2 - l1*m_l3*sin(pi/2)*cos(q(2))*sin(q(1)) - (l2*m_l3*sin(pi/2)*cos(q(2))*sin(q(1)))/2 + l1*m_l3*cos(pi/2)*sin(pi/2)*sin(q(2)) + (l2*m_l3*cos(pi/2)*sin(pi/2)*sin(q(2)))/2 - l1*m_l3*cos(pi/2)*sin(pi/2)*cos(q(1))*sin(q(2)) - (l2*m_l3*cos(pi/2)*sin(pi/2)*cos(q(1))*sin(q(2)))/2) - g*sin(phi)*sin(theta)*(m_l3*(l1 + l2/2)*(sin(q(2)) - cos(pi/2)^2*sin(q(2)) + cos(pi/2)*cos(q(2))*sin(q(1)) + cos(pi/2)^2*cos(q(1))*sin(q(2))) + (l1*m_l2*cos(pi/2)*sin(q(1)))/2);
% g_phib(3) = 0;


% Derivative of U wrt q
% U_manip = sum(m_li * g * e3' * R_b * p_b_li)
% derivative(p_b_li) = J_P_li
sum_m = (m_l1 * J_P_l1 + m_l2 * J_P_l2 + m_l3 * J_P_l3);
% g_q = (g * e3' * R_b * sum_m)';
g_q = (g * e3' * sum_m)';

% Full g vector
% g_vector = [g_pb; g_phib; g_q];
g_vector = g_q;

%% Coriolis matrix C(csi, csi_dot) (using Christoffel symbols of the first type)
% Computed using external script
C = calculate_C_matrix_manipulator(q, q_dot, m_l1, m_l2, m_l3, l1, l2, offset, H_l1, H_l2, H_l3, pi);

%% Forces applied to manipulator
torque_q = u + u_ext - C * q_dot - g_vector;        % torques applied to the joints

% Static
% u = J' * w
pseudo = J_e_e * inv(J_e_e' * J_e_e);
w_e_e = pseudo * torque_q;                          % end-effector wrench

%% Generelized vector acceleration
% B * csi_ddot + C * csi_dot + g = u + u_ext
% q_ddot = B \ (u + u_ext - C * q_dot - g_vector);
q_ddot = B \ torque_q;

end

function S = skew(v)
    if(numel(v)~= 1)
        S= [0 -v(3) v(2); 
            v(3) 0 -v(1);
            -v(2) v(1) 0];
    else
        S= zeros(3);
    end
end

== matlab function UAM_decentralized/Wrench Transformation ==
  data: w_uav input; manipulator_effect output; w_e_e input; uav_effect output; R_b_e input; p_b_e input
function [manipulator_effect,uav_effect] = fcn(w_uav, w_e_e, R_b_e, p_b_e)
% The Passivity based Control needs the z-axis pointing downward
% The Impedence Control needs the z-axis pointing upward
% Rotation between the frame used in the Passivity based Control and the frame used in the Impedence Control

% Rotation about X-axis
R_pass_imp = [  1,  0,          0;
                0,  cos(pi),    -sin(pi);
                0,  sin(pi),    cos(pi)];

%% UAV Effect on the end-effector of the manipulator
% Force transformation between two frames
% w_1 = [R_1_2                  zeros(3,3);
%        skew(r_1_2)*R_1_2      R_1_2]      * w_2

R_e_uav = (R_pass_imp * R_b_e)';
r_e_uav = - R_b_e' * p_b_e;     % expressed in end-effector frame
uav_effect = [  R_e_uav                 zeros(3,3);
                skew(r_e_uav)*R_e_uav   R_e_uav]    * w_uav;


%% Manipulator Effect on the UAV
% Force transformation between two frames
% w_1 = [R_1_2                  zeros(3,3);
%        skew(r_1_2)*R_1_2      R_1_2]      * w_2

r_uav_e = R_pass_imp * p_b_e;

J_pass_e = [R_e_uav'                        zeros(3,3);
            skew(r_uav_e) * R_e_uav'        R_e_uav'];

manipulator_effect = J_pass_e * w_e_e;

end
function S = skew(v)
    if(numel(v)~= 1)
        S= [0 -v(3) v(2); 
            v(3) 0 -v(1);
            -v(2) v(1) 0];
    else
        S= zeros(3);
    end
end

== matlab function UAM_decentralized/MATLAB Function1 ==
  data: f_ext input; J input; u_ext output
function u_ext = fcn(f_ext, J)

u_ext = J' * f_ext;

== matlab function UAM_decentralized/MATLAB Function5 ==
  data: u input; norma output
function norma = fcn(u)
norma = norm([u(1);u(2);u(3)]);

== matlab function UAM_decentralized/determinant ==
  data: u input; y output
function y = fcn(u)

y = det(u);

== matlab function UAM_decentralized/MATLAB Function6 ==
  data: u input; norma output
function norma = fcn(u)
norma = norm([u(1);u(2);u(3)]);

== matlab function UAM_decentralized/MATLAB Function2 ==
  data: u input; norma output
function norma = fcn(u)
norma = norm([u(1);u(2);u(3)]);

== matlab function UAM_decentralized/Cartesian Impedance Control ==
  data: x_d_ddot input; u output; x_d_dot input; x_tilde_dot input; x_tilde input; J input; J_dot input; B input; C input; g_vector input
function u = fcn(x_d_ddot, x_d_dot, x_tilde_dot, x_tilde, J,J_dot, B,C,g_vector)

%% Case study A - Rigid Behavior
% Kp = 80 * eye(3);
% zeta = 0.8 * ones(3,1);

%% Case study A - Compliant Behavior
% Kp = 10 * eye(3);
% zeta = 0.5 * ones(3,1);

%% Case study B
Kp = 100*eye(3);
zeta = zeros(3,1);                 % Damping ratio
zeta(1:3) = 0.85;

%% Control
Kd = zeros(3,3);
for i=1:3
    Kd(i,i) = 2 * zeta(i) * sqrt(Kp(i,i)); 
end

inv_J = inv(J);
Bx = inv_J' * B * inv_J;
Cx = inv_J' * (C - B * inv_J * J_dot) * inv_J;

u = g_vector + J' * (Bx * x_d_ddot + Cx * x_d_dot + Kd * x_tilde_dot + Kp * x_tilde);

== matlab function UAM_decentralized/UAV/UAV dynamics ==
  data: force_b output; torque_b output; uT input; p_b_ddot output; tau_b_b input; f_b_ext input; tau_b_ext input; f_wind input; eta_b input; eta_b_dot input; eta_b_ddot output; m_b parameter; H_b parameter
function [force_b,torque_b,  p_b_ddot, eta_b_ddot] = fcn(uT,tau_b_b,  f_b_ext, tau_b_ext, f_wind,  eta_b, eta_b_dot,  m_b,H_b)

% parameters
g = 9.81;
e3 = [0;0;1];

%% Extracting variables
% Euler angles
phi = eta_b(1);    % Roll angle
theta = eta_b(2);  % Pitch angle
psi = eta_b(3);    % Yaw angle

phi_dot = eta_b_dot(1);   
theta_dot = eta_b_dot(2);  
%psi_dot = eta_b_dot(3);    

%% Mapping between squared propellers speed omega_i^2 and control wrench [f_b; tau_b_b]
% w_b = Allocation_matrix * [omega1^2; omega2^2; omega3^2; omega4^2];     % control wrench
% uT = w_b(3);        % total thrust
% tau_b_b = w_b(4:6);   % control torques (in the body frame)

%% Rotation Matrices and Angular Velocity Mapping
% Individual Rotation Matrices
% Rotation about X-axis (Roll)
Rx = [1,           0,          0;
      0, cos(phi), -sin(phi);
      0, sin(phi),  cos(phi)];

% Rotation about Y-axis (Pitch)
Ry = [cos(theta),  0, sin(theta);
      0,           1,          0;
     -sin(theta),  0, cos(theta)];

% Rotation about Z-axis (Yaw)
Rz = [cos(psi), -sin(psi), 0;
      sin(psi),  cos(psi), 0;
      0,         0,         1];

% Combined Rotation Matrix R_b (from UAV body frame to Inertial frame)
% Using Z-Y-X Euler angle convention (Yaw-Pitch-Roll)
R_b = Rz * Ry * Rx;

% mapping between time derivative of eta_b into UAV angular velocity omega_b_b expressed wrt Sigma_b
Q = [   1     0           -sin(theta);
        0     cos(phi)    cos(theta)*sin(phi);
        0     -sin(phi)   cos(theta)*cos(phi)];

Q_dot = [ 0,     0,                     -cos(theta)*theta_dot;
          0,    -sin(phi)*phi_dot,     -sin(theta)*sin(phi)*theta_dot + cos(theta)*cos(phi)*phi_dot;
          0,    -cos(phi)*phi_dot,     -sin(theta)*cos(phi)*theta_dot - cos(theta)*sin(phi)*phi_dot ];

%% Dynamic Matrices
M = Q' * H_b * Q;    % inertia matrix
C = Q' * skew(Q * eta_b_dot) * H_b * Q + Q' * H_b * Q_dot;    % Coriolis matrix

%% Forces applied to the UAV
force = m_b * g * e3 - uT * R_b * e3 + R_b * f_b_ext + f_wind;         % expressed in the inertial frame
torque = -C * eta_b_dot + Q' * tau_b_b + Q' * tau_b_ext;

force_b = R_b' * force;                             % espressed in the body frame
torque_b = Q' * torque;

%% Accelerations
% p_b_ddot = 1/m_b * (m_b * g * e3 - uT * R_b * e3 + f_e);
% eta_b_ddot = M \ (-C * eta_b_dot + Q' * tau_b_b + tau_e);

p_b_ddot = 1/m_b * force;
eta_b_ddot = M \ torque;

end

function S = skew(v)
if(numel(v)~= 1)
S= [0 -v(3) v(2); 
    v(3) 0 -v(1);
    -v(2) v(1) 0];
else
S= zeros(3);
end
end

== matlab function UAM_decentralized/Attitude passive controller ==
  data: eta_d input; tau_b_b output; eta_d_dot input; eta_d_ddot input; eta_b input; eta_b_dot input; tau_e_hat input; H_b parameter
function tau_b_b = fcn(eta_d, eta_d_dot, eta_d_ddot,  eta_b, eta_b_dot,  tau_e_hat, H_b)
%% Case study A - Rigid Behavior
% K_o = 80 * eye(3);
% zeta = 0.8;

%% Case study A - Compliant Behavior
% K_o = 50 * eye(3); %5
% zeta = 0.5;

%% Case study B
K_o = 50 * eye(3);
zeta = 0.5;

%% Gain matrices
D_o = zeros(3,3);
for i=1:3
    D_o(i,i) = 2 * zeta * sqrt(K_o(i,i)); 
end
%% GAINS
% K_o = 80*eye(3);
% D_o = 20*eye(3);

%% INNER LOOP ATTITUDE CONTROL
ni = K_o(1,1)/D_o(1,1);     % coupling parameter > 0

% Getting the state variables
phi = eta_b(1);
theta = eta_b(2);
phi_dot = eta_b_dot(1);
theta_dot = eta_b_dot(2);

Q = [   1,   0,         -sin(theta);
        0,   cos(phi),  cos(theta)*sin(phi);
        0,  -sin(phi), cos(theta)*cos(phi) ];

Q_dot = [0        0                 cos(theta)*theta_dot;
         0    -sin(phi)*phi_dot    -sin(theta)*theta_dot*sin(phi) + cos(theta)*cos(phi)*phi_dot;
         0    -cos(phi)*phi_dot    -sin(theta)*theta_dot*cos(phi) - cos(theta)*sin(phi)*phi_dot];

% Inertia and Coriolis matrices M and C
M = Q' * H_b * Q;
C = Q' * skew(Q * eta_b_dot) * H_b * Q + Q' * H_b * Q_dot;

e_eta = eta_b - eta_d;                      % angular tracking error
e_eta_dot = eta_b_dot - eta_d_dot;

eta_r_dot = eta_d_dot - ni * e_eta;         % reference vector for the attitude velocity
eta_r_ddot = eta_d_ddot - ni * e_eta_dot;

ni_eta = e_eta_dot + ni * e_eta;

tau_b_b = Q' \ (M * eta_r_ddot + C * eta_r_dot - tau_e_hat - D_o * ni_eta - K_o * e_eta);

end

function S = skew(v)
if(numel(v)~= 1)
S= [0 -v(3) v(2); 
    v(3) 0 -v(1);
    -v(2) v(1) 0];
else
S= zeros(3);
end
end

== matlab function UAM_decentralized/Position passive controller ==
  data: p_d input; mu_d output; p_d_dot input; p_d_ddot input; p_b input; p_b_dot input; m_b parameter
function mu_d = fcn(p_d, p_d_dot, p_d_ddot, p_b, p_b_dot,m_b)
% Compute the virtual control input based on position error
% eq 19

%% GAINS
%% Case study A - Rigid Behavior
% K_p = 10 * eye(3);
% zeta = 0.8;

%% Case study A - Compliant Behavior
% K_p = 10 * eye(3); %5
% zeta = 0.5;

%% Case study B
K_p = 10 * eye(3);
zeta = 0.5;
%% Gain matrices
D_p = zeros(3,3);
for i=1:3
    D_p(i,i) = 2 * zeta * sqrt(K_p(i,i)); 
end
% K_p = 10*eye(3);
% D_p = diag([10, 10, 10]);

%% OUTER LOOP POSITION CONTROL
% Position and velocity errors
e_p = p_b - p_d;
e_p_dot = p_b_dot - p_d_dot;

% Virtual control input (mu_d)
mu_d = p_d_ddot -  (D_p * e_p_dot + K_p * e_p);
% mu_d = p_d_ddot - (1/m_b) * (D_p * e_p_dot + K_p * e_p);
end

== matlab function UAM_decentralized/Thrust and Attitude references/Thrust and attitude references not filtered ==
  data: mu_d input; uT output; f_e_hat input; psi_d input; eta_d output; m_b parameter
function [uT, eta_d] = fcn(mu_d, f_e_hat, psi_d,m_b)
% Compute total thrust and desired attitude from the virtual control input
% Eq 21

% Parameters
g = 9.81; 

% Modified virtual input
mu_bar = mu_d - (1/m_b) * f_e_hat;

% Extract components of mu_bar
mu_bar_1 = mu_bar(1);
mu_bar_2 = mu_bar(2);
mu_bar_3 = mu_bar(3);

% Total Thrust
% Eq. 21a
uT = m_b * sqrt(mu_bar_1^2 + mu_bar_2^2 + (mu_bar_3 - g)^2);

% Eq 21b
phi_d = asin(m_b/uT * (mu_bar_2 * cos(psi_d) - mu_bar_1 * sin(psi_d)));

% Eq 21c
theta_d = atan((mu_bar_1 * cos(psi_d) + mu_bar_2 * sin(psi_d)) / (mu_bar_3 - g));

% Desired attitude vector
eta_d = [phi_d; theta_d; psi_d];

end
